simulink model "PVarray_Grid_IncCondReg_det"  (Simulink 8.3)
settings: Solver=FixedStepDiscrete  SolverMode=SingleTasking  StartTime=0.0  StopTime=0.5  RelTol=1e-3
PreLoadFcn:
  | Ts_Power=1e-6
  | Ts_Control=100e-6
undefined symbols (not defined in the file): D1, Delta, DiscIntNeverNeededParam, level, sigbuilder_block
libraries: powerlib x30, powerlib_extras x8, simulink x4
(part 2 of 2)

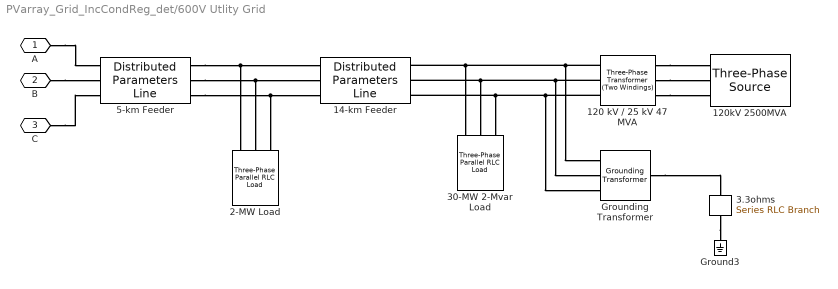
== system PVarray_Grid_IncCondReg_det/600V Utlity Grid ==
  120 kV / 25 kV 47 MVA : powerlib/Elements/Three-Phase Transformer (Two Windings)  Winding1Connection=Yg  UNITS=pu  NominalPower=[47e6 60 ]  Winding1="[ 120e3  0.08/30   0.08 ]"  Winding2Connection=Delta (D1)  Winding2="[ 25e3  0.08/30  0.08]"  SetSaturation=off  Rm=500  Lm=500  Saturation="[ 0,0  ;  0.005,1.2  ;  1.0,1.4 ]"  Hysteresis=off  DataFile='basic_model'  SetInitialFlux=off  InitialFluxes=[ 0.8 , -0.8 , 0.7 ]  Measurements=None  MoreParameters=off  BreakLoop=off  DataType=off  TransfoNumber=0
  120kV 2500MVA : powerlib/Electrical Sources/Three-Phase Source  Voltage=120e3  PhaseAngle=0  Frequency=60  InternalConnection=Yg  SpecifyImpedance=on  Resistance=0.8929  Inductance=16.58e-3  ShortCircuitLevel=2500e6  BaseVoltage=120e3  XRratio=7  BusType=swing  Pref=0  Qref=0  Qmin=-inf  Qmax=inf
  14-km Feeder : powerlib/Elements/Distributed Parameters Line  Phases=3  Frequency=60  Resistance=[0.1153 0.413]  Inductance=[1.05e-3 3.32e-3]  Capacitance=[11.33e-009 5.01e-009]  Length=14  x1=[-5.8e-05 1.17635592444979e-09 0 0;-5.7e-05 1.1770598483649e-09 0 0;-5.6e-05 1.17776360499355e-09 0 0;-5.5e-05 1.17846719423573e-09 0 0;-5.4e-05 1.17917061599144e-09 0 0;-5.3e-05 1.17987387016071e-09 0 0;-5.2e-05 1.18057695664358e-09 0 0;-5.1e-05 1.18127987534014e-09 0 0;-5e-05 1.18198262615049e-09 0 0;-4.9e-05 1.18268520897475e-09 -3790.50088209165 -24060.9143986541;-4.8e-05 1.18338762371306e-09 -3781.42986191954 -24062.3416739909;-4.7e-05 1.1840898702656e-09 -3772.35830432192 -24063.7655295324;-4.6e-05 1.18479194853256e-09 -3763.28621058805 -24065.1859650761;-4.5e-05 1.18549385841416e-09 -3754.21358200728 -24066.6029804202;-4.4e-05 1.18619559981065e-09 -3745.14041986903 -24068.0165753633;-4.3e-05 1.18689717262229e-09 -3736.06672546281 -24069.4267497044;-4.2e-05 1.18759857674937e-09 -3726.99250007819 -24070.8335032433;-4.1e-05 1.1882998120922e-09 -3717.91774500481 -24072.2368357798;-4e-05 1.18900087855114e-09 -3708.84246153241 -24073.6367471147;-3.9e-05 1.18970177602653e-09 -3699.76665095078 -24075.0332370489;-3.8e-05 1.19040250441876e-09 -3690.6903145498 -24076.426305384;-3.7e-05 1.19110306362825e-09 -3681.61345361941 -24077.8159519219;-3.6e-05 1.19180345355544e-09 -3672.53606944965 -24079.2021764653;-3.5e-05 1.19250367410077e-09 -3663.45816333061 -24080.584978817;-3.4e-05 1.19320372516474e-09 -3654.37973655246 -24081.9643587805;-3.3e-05 1.19390360664784e-09 -3645.30079040545 -24083.3403161598;-3.2e-05 1.19460331845062e-09 -3636.22132617991 -24084.7128507594;-3.1e-05 1.19530286047362e-09 -3627.14134516621 -24086.0819623841;-3e-05 1.19600223261744e-09 -3618.06084865485 -24087.4476508394;-2.9e-05 1.19670143478266e-09 -3608.97983793634 -24088.8099159313;-2.8e-05 1.19740046686991e-09 -3599.89831430132 -24090.168757466;-2.7e-05 1.19809932877986e-09 -3590.81627904046 -24091.5241752505;-2.6e-05 1.19879802041318e-09 -3581.73373344453 -24092.8761690921;-2.5e-05 1.19949654167056e-09 -3572.65067880435 -24094.2247387987;-2.4e-05 1.20019489245273e-09 -3563.56711641084 -24095.5698841786;-2.3e-05 1.20089307266044e-09 -3554.48304755497 -24096.9116050407;-2.2e-05 1.20159108219446e-09 -3545.39847352778 -24098.2499011942;-2.1e-05 1.20228892095559e-09 -3536.3133956204 -24099.584772449;-2e-05 1.20298658884465e-09 -3527.22781512403 -24100.9162186153;-1.9e-05 1.20368408576249e-09 -3518.14173332992 -24102.244239504;-1.8e-05 1.20438141160998e-09 -3509.0551515294 -24103.5688349262;-1.7e-05 1.20507856628801e-09 -3499.96807101389 -24104.8900046937;-1.6e-05 1.2057755496975e-09 -3490.88049307487 -24106.2077486188;-1.5e-05 1.20647236173939e-09 -3481.79241900387 -24107.5220665142;-1.4e-05 1.20716900231466e-09 -3472.70385009252 -24108.832958193;-1.3e-05 1.20786547132428e-09 -3463.61478763251 -24110.140423469;-1.2e-05 1.20856176866929e-09 -3454.52523291559 -24111.4444621563;-1.1e-05 1.20925789425071e-09 -3445.43518723359 -24112.7450740697;-1e-05 1.20995384796962e-09 -3436.34465187842 -24114.0422590242;-9e-06 1.21064962972711e-09 -3427.25362814203 -24115.3360168356;-8e-06 1.21134523942428e-09 -3418.16211731647 -24116.6263473199;-7e-06 1.21204067696228e-09 -3409.07012069384 -24117.9132502937;-6e-06 1.21273594224227e-09 -3399.97763956632 -24119.1967255742;-5e-06 1.21343103516543e-09 -3390.88467522615 -24120.476772979;-4e-06 1.21412595563299e-09 -3381.79122896565 -24121.753392326;-3e-06 1.21482070354617e-09 -3372.69730207719 -24123.026583434;-2e-06 1.21551527880623e-09 -3363.60289585323 -24124.2963461219;-1e-06 1.21620968131446e-09 -3354.50801158628 -24125.5626802092]  x2=[-5.8e-05 1.27313609791547e-09 0 0;-5.7e-05 1.27386533401627e-09 0 0;-5.6e-05 1.27459438907241e-09 0 0;-5.5e-05 1.27532326298026e-09 0 0;-5.4e-05 1.27605195563622e-09 0 0;-5.3e-05 1.27678046693675e-09 0 0;-5.2e-05 1.2775087967783e-09 0 0;-5.1e-05 1.27823694505736e-09 0 0;-5e-05 1.27896491167044e-09 0 0;-4.9e-05 1.27969269651409e-09 -3379.3379853252 -24243.9018981791;-4.8e-05 1.28042029948486e-09 -3370.19800971033 -24245.174155756;-4.7e-05 1.28114772047935e-09 -3361.05755511516 -24246.4429675529;-4.6e-05 1.28187495939418e-09 -3351.91662283875 -24247.7083333896;-4.5e-05 1.28260201612599e-09 -3342.77521418024 -24248.9702530861;-4.4e-05 1.28332889057145e-09 -3333.63333043882 -24250.2287264632;-4.3e-05 1.28405558262726e-09 -3324.49097291376 -24251.483753342;-4.2e-05 1.28478209219012e-09 -3315.34814290439 -24252.735333544;-4.1e-05 1.28550841915681e-09 -3306.20484171011 -24253.9834668915;-4e-05 1.28623456342407e-09 -3297.06107063039 -24255.228153207;-3.9e-05 1.28696052488872e-09 -3287.91683096476 -24256.4693923137;-3.8e-05 1.28768630344758e-09 -3278.77212401283 -24257.7071840352;-3.7e-05 1.28841189899749e-09 -3269.62695107425 -24258.9415281954;-3.6e-05 1.28913731143534e-09 -3260.48131344876 -24260.172424619;-3.5e-05 1.28986254065803e-09 -3251.33521243617 -24261.3998731311;-3.4e-05 1.29058758656249e-09 -3242.18864933633 -24262.6238735572;-3.3e-05 1.29131244904567e-09 -3233.04162544918 -24263.8444257234;-3.2e-05 1.29203712800455e-09 -3223.89414207471 -24265.0615294561;-3.1e-05 1.29276162333614e-09 -3214.74620051298 -24266.2751845825;-3e-05 1.29348593493747e-09 -3205.59780206413 -24267.4853909299;-2.9e-05 1.2942100627056e-09 -3196.44894802833 -24268.6921483265;-2.8e-05 1.29493400653762e-09 -3187.29963970586 -24269.8954566007;-2.7e-05 1.29565776633064e-09 -3178.14987839702 -24271.0953155815;-2.6e-05 1.2963813419818e-09 -3168.99966540221 -24272.2917250983;-2.5e-05 1.29710473338825e-09 -3159.84900202187 -24273.4846849812;-2.4e-05 1.2978279404472e-09 -3150.69788955652 -24274.6741950606;-2.3e-05 1.29855096305585e-09 -3141.54632930674 -24275.8602551674;-2.2e-05 1.29927380111145e-09 -3132.39432257315 -24277.042865133;-2.1e-05 1.29999645451126e-09 -3123.24187065648 -24278.2220247895;-2e-05 1.30071892315259e-09 -3114.08897485748 -24279.3977339692;-1.9e-05 1.30144120693275e-09 -3104.93563647699 -24280.5699925049;-1.8e-05 1.30216330574909e-09 -3095.78185681591 -24281.7388002302;-1.7e-05 1.30288521949899e-09 -3086.62763717517 -24282.9041569789;-1.6e-05 1.30360694807983e-09 -3077.47297885582 -24284.0660625853;-1.5e-05 1.30432849138906e-09 -3068.31788315892 -24285.2245168844;-1.4e-05 1.30504984932412e-09 -3059.16235138562 -24286.3795197115;-1.3e-05 1.3057710217825e-09 -3050.00638483713 -24287.5310709024;-1.2e-05 1.30649200866169e-09 -3040.84998481471 -24288.6791702935;-1.1e-05 1.30721280985922e-09 -3031.69315261969 -24289.8238177216;-1e-05 1.30793342527267e-09 -3022.53588955346 -24290.965013024;-9e-06 1.3086538547996e-09 -3013.37819691747 -24292.1027560386;-8e-06 1.30937409833764e-09 -3004.22007601324 -24293.2370466037;-7e-06 1.31009415578442e-09 -2995.06152814233 -24294.3678845579;-6e-06 1.3108140270376e-09 -2985.90255460639 -24295.4952697407;-5e-06 1.31153371199487e-09 -2976.74315670711 -24296.6192019918;-4e-06 1.31225321055396e-09 -2967.58333574623 -24297.7396811514;-3e-06 1.31297252261259e-09 -2958.42309302558 -24298.8567070603;-2e-06 1.31369164806855e-09 -2949.26242984704 -24299.9702795598;-1e-06 1.31441058681963e-09 -2940.10134751252 -24301.0803984916]  x3=[-5.8e-05 -2.75037560687932e-13 0 0;-5.7e-05 -2.71761263610655e-13 0 0;-5.6e-05 -2.68484927910041e-13 0 0;-5.5e-05 -2.65208554051731e-13 0 0;-5.4e-05 -2.61932142501371e-13 0 0;-5.3e-05 -2.58655693724612e-13 0 0;-5.2e-05 -2.55379208187111e-13 0 0;-5.1e-05 -2.52102686354528e-13 0 0;-5e-05 -2.48826128692532e-13 0 0;-4.9e-05 -2.45549535666793e-13 -23.6102100345883 -155.666879550902;-4.8e-05 -2.4227290774299e-13 -23.5515233271852 -155.675769328311;-4.7e-05 -2.38996245386803e-13 -23.4928332725853 -155.684636980721;-4.6e-05 -2.35719549063919e-13 -23.43413987913 -155.693482506872;-4.5e-05 -2.32442819240031e-13 -23.3754431551607 -155.702305905508;-4.4e-05 -2.29166056380834e-13 -23.3167431090196 -155.711107175373;-4.3e-05 -2.2588926095203e-13 -23.2580397490494 -155.719886315217;-4.2e-05 -2.22612433419324e-13 -23.199333083593 -155.728643323792;-4.1e-05 -2.19335574248427e-13 -23.140623120994 -155.737378199855;-4e-05 -2.16058683905053e-13 -23.0819098695963 -155.746090942162;-3.9e-05 -2.12781762854921e-13 -23.0231933377445 -155.754781549477;-3.8e-05 -2.09504811563756e-13 -22.9644735337835 -155.763450020564;-3.7e-05 -2.06227830497284e-13 -22.9057504660586 -155.77209635419;-3.6e-05 -2.02950820121239e-13 -22.8470241429158 -155.780720549128;-3.5e-05 -1.99673780901356e-13 -22.7882945727013 -155.789322604151;-3.4e-05 -1.96396713303376e-13 -22.7295617637619 -155.797902518037;-3.3e-05 -1.93119617793042e-13 -22.6708257244449 -155.806460289567;-3.2e-05 -1.89842494836105e-13 -22.612086463098 -155.814995917523;-3.1e-05 -1.86565344898314e-13 -22.5533439880693 -155.823509400694;-3e-05 -1.83288168445428e-13 -22.4945983077074 -155.832000737869;-2.9e-05 -1.80010965943205e-13 -22.4358494303615 -155.840469927842;-2.8e-05 -1.7673373785741e-13 -22.3770973643809 -155.848916969408;-2.7e-05 -1.73456484653808e-13 -22.3183421181158 -155.857341861368;-2.6e-05 -1.70179206798172e-13 -22.2595836999166 -155.865744602523;-2.5e-05 -1.66901904756276e-13 -22.200822118134 -155.87412519168;-2.4e-05 -1.63624578993896e-13 -22.1420573811196 -155.882483627647;-2.3e-05 -1.60347229976815e-13 -22.083289497225 -155.890819909237;-2.2e-05 -1.57069858170816e-13 -22.0245184748024 -155.899134035265;-2.1e-05 -1.53792464041688e-13 -21.9657443222046 -155.907426004549;-2e-05 -1.5051504805522e-13 -21.9069670477846 -155.915695815911;-1.9e-05 -1.47237610677208e-13 -21.8481866598961 -155.923943468176;-1.8e-05 -1.43960152373447e-13 -21.789403166893 -155.93216896017;-1.7e-05 -1.40682673609739e-13 -21.7306165771297 -155.940372290726;-1.6e-05 -1.37405174851884e-13 -21.6718268989613 -155.948553458677;-1.5e-05 -1.3412765656569e-13 -21.6130341407428 -155.956712462861;-1.4e-05 -1.30850119216965e-13 -21.5542383108303 -155.964849302118;-1.3e-05 -1.2757256327152e-13 -21.4954394175798 -155.972963975292;-1.2e-05 -1.24294989195168e-13 -21.4366374693479 -155.981056481229;-1.1e-05 -1.21017397453727e-13 -21.3778324744918 -155.989126818779;-1e-05 -1.17739788513014e-13 -21.3190244413689 -155.997174986795;-9e-06 -1.14462162838852e-13 -21.2602133783372 -156.005200984134;-8e-06 -1.11184520897063e-13 -21.2013992937551 -156.013204809655;-7e-06 -1.07906863153475e-13 -21.1425821959813 -156.02118646222;-6e-06 -1.04629190073915e-13 -21.083762093375 -156.029145940694;-5e-06 -1.01351502124213e-13 -21.0249389942959 -156.037083243948;-4e-06 -9.80737997702028e-14 -20.9661129071042 -156.044998370852;-3e-06 -9.47960834777184e-14 -20.9072838401601 -156.052891320281;-2e-06 -9.15183537125964e-14 -20.8484518018248 -156.060762091115;-1e-06 -8.82406109406753e-14 -20.7896168004596 -156.068610682234]  x4=[-5.8e-05 3.5411822113335e-12 0 0;-5.7e-05 3.53990398331012e-12 0 0;-5.6e-05 3.53862525218744e-12 0 0;-5.5e-05 3.53734601814719e-12 0 0;-5.4e-05 3.53606628137119e-12 0 0;-5.3e-05 3.53478604204131e-12 0 0;-5.2e-05 3.53350530033949e-12 0 0;-5.1e-05 3.53222405644777e-12 0 0;-5e-05 3.53094231054824e-12 0 0;-4.9e-05 3.52966006282306e-12 -1.28892375629158 -2.1654706090284;-4.8e-05 3.52837731345447e-12 -1.28810730153168 -2.16595636794452;-4.7e-05 3.52709406262477e-12 -1.28729066370301 -2.16644181902993;-4.6e-05 3.52581031051635e-12 -1.28647384292163 -2.16692696221564;-4.5e-05 3.52452605731165e-12 -1.28565683930363 -2.16741179743271;-4.4e-05 3.52324130319319e-12 -1.28483965296511 -2.16789632461222;-4.3e-05 3.52195604834357e-12 -1.28402228402223 -2.16838054368532;-4.2e-05 3.52067029294545e-12 -1.28320473259114 -2.16886445458318;-4.1e-05 3.51938403718157e-12 -1.28238699878805 -2.16934805723704;-4e-05 3.51809728123472e-12 -1.28156908272916 -2.16983135157815;-3.9e-05 3.5168100252878e-12 -1.28075098453072 -2.17031433753784;-3.8e-05 3.51552226952373e-12 -1.27993270430901 -2.17079701504747;-3.7e-05 3.51423401412555e-12 -1.27911424218031 -2.17127938403842;-3.6e-05 3.51294525927635e-12 -1.27829559826096 -2.17176144444215;-3.5e-05 3.51165600515927e-12 -1.27747677266729 -2.17224319619014;-3.4e-05 3.51036625195756e-12 -1.27665776551568 -2.17272463921393;-3.3e-05 3.50907599985453e-12 -1.27583857692254 -2.1732057734451;-3.2e-05 3.50778524903353e-12 -1.27501920700427 -2.17368659881526;-3.1e-05 3.50649399967802e-12 -1.27419965587735 -2.17416711525607;-3e-05 3.50520225197151e-12 -1.27337992365823 -2.17464732269925;-2.9e-05 3.50391000609759e-12 -1.27256001046343 -2.17512722107655;-2.8e-05 3.50261726223992e-12 -1.27173991640947 -2.17560681031976;-2.7e-05 3.50132402058221e-12 -1.27091964161291 -2.17608609036072;-2.6e-05 3.50003028130828e-12 -1.27009918619032 -2.17656506113132;-2.5e-05 3.49873604460199e-12 -1.26927855025831 -2.17704372256348;-2.4e-05 3.49744131064728e-12 -1.26845773393352 -2.17752207458918;-2.3e-05 3.49614607962816e-12 -1.26763673733259 -2.17800011714043;-2.2e-05 3.49485035172872e-12 -1.26681556057221 -2.17847785014929;-2.1e-05 3.49355412713309e-12 -1.26599420376909 -2.17895527354786;-2e-05 3.49225740602552e-12 -1.26517266703995 -2.1794323872683;-1.9e-05 3.49096018859028e-12 -1.26435095050157 -2.17990919124279;-1.8e-05 3.48966247501174e-12 -1.26352905427072 -2.18038568540356;-1.7e-05 3.48836426547434e-12 -1.26270697846421 -2.1808618696829;-1.6e-05 3.48706556016259e-12 -1.26188472319888 -2.18133774401314;-1.5e-05 3.48576635926105e-12 -1.26106228859158 -2.18181330832663;-1.4e-05 3.48446666295437e-12 -1.26023967475922 -2.1822885625558;-1.3e-05 3.48316647142727e-12 -1.25941688181868 -2.18276350663309;-1.2e-05 3.48186578486453e-12 -1.25859390988693 -2.183238140491;-1.1e-05 3.48056460345102e-12 -1.25777075908091 -2.18371246406209;-1e-05 3.47926292737165e-12 -1.25694742951761 -2.18418647727894;-9e-06 3.47796075681142e-12 -1.25612392131405 -2.18466018007417;-8e-06 3.47665809195541e-12 -1.25530023458727 -2.18513357238048;-7e-06 3.47535493298875e-12 -1.25447636945433 -2.18560665413057;-6e-06 3.47405128009665e-12 -1.25365232603233 -2.18607942525721;-5e-06 3.47274713346438e-12 -1.25282810443836 -2.18655188569321;-4e-06 3.47144249327729e-12 -1.25200370478959 -2.18702403537143;-3e-06 3.47013735972081e-12 -1.25117912720316 -2.18749587422476;-2e-06 3.46883173298042e-12 -1.25035437179628 -2.18796740218613;-1e-06 3.46752561324168e-12 -1.24952943868616 -2.18843861918855]  x5=5.70973484498186e-05  V1=ones(3,3)  V2=ones(3,3)  I1=ones(3,3)  I2=ones(3,3)  nHarmo=1  Measurements=None
  2-MW Load : powerlib/Elements/Three-Phase Parallel RLC Load  LConnTagsString=A|B|C  Configuration=Y (grounded)  NominalVoltage=25e3  NominalFrequency=60  ActivePower=2e6  InductivePower=0  CapacitivePower=0  Measurements=None  LoadType=constant Z
  "3.3ohms " : powerlib/Elements/Series RLC Branch  LConnTagsString=__new0  RConnTagsString=__new0  BranchType=R  Resistance=3.3  Inductance=[]  SetiL0=off  InitialCurrent=0  Capacitance=[]  Setx0=off  InitialVoltage=0  Measurements=None
  30-MW 2-Mvar Load : powerlib/Elements/Three-Phase Parallel RLC Load  LConnTagsString=A|B|C  Configuration=Y (grounded)  NominalVoltage=25e3  NominalFrequency=60  ActivePower=30e6  InductivePower=2e6  CapacitivePower=0  Measurements=None  LoadType=constant Z
  5-km Feeder : powerlib/Elements/Distributed Parameters Line  Phases=3  Frequency=60  Resistance=[0.1153 0.413]  Inductance=[1.05e-3 3.32e-3]  Capacitance=[11.33e-009 5.01e-009]  Length=5  x1=[-2.1e-05 1.20806252804395e-09 -3536.88834563418 -24100.7824567799;-2e-05 1.2087451259397e-09 -3527.8023135806 -24102.1141196122;-1.9e-05 1.2094275520458e-09 -3518.71578014764 -24103.4423569965;-1.8e-05 1.21010980626528e-09 -3509.62874662669 -24104.7671687441;-1.7e-05 1.21079188850117e-09 -3500.54121430922 -24106.0885546668;-1.6e-05 1.21147379865653e-09 -3491.45318448679 -24107.4065145766;-1.5e-05 1.21215553663444e-09 -3482.36465845099 -24108.7210482863;-1.4e-05 1.21283710233802e-09 -3473.2756374935 -24110.0321556092;-1.3e-05 1.2135184956704e-09 -3464.18612290609 -24111.3398363587;-1.2e-05 1.21419971653473e-09 -3455.09611598058 -24112.6440903491;-1.1e-05 1.21488076483421e-09 -3446.00561800885 -24113.9449173951;-1e-05 1.21556164047204e-09 -3436.91463028287 -24115.2423173117;-9e-06 1.21624234335145e-09 -3427.82315409468 -24116.5362899146;-8e-06 1.21692287337569e-09 -3418.73119073637 -24117.8268350198;-7e-06 1.21760323044806e-09 -3409.63874150011 -24119.1139524439;-6e-06 1.21828341447186e-09 -3400.54580767814 -24120.3976420041;-5e-06 1.21896342535041e-09 -3391.45239056278 -24121.6779035178;-4e-06 1.21964326298707e-09 -3382.3584914464 -24122.9547368032;-3e-06 1.22032292728523e-09 -3373.26411162145 -24124.2281416787;-2e-06 1.22100241814828e-09 -3364.16925238043 -24125.4981179633;-1e-06 1.22168173547966e-09 -3355.07391501594 -24126.7646654767]  x2=[-2.1e-05 1.20229252106794e-09 -3536.3133956204 -24099.584772449;-2e-05 1.20299001752641e-09 -3527.22781512403 -24100.9162186153;-1.9e-05 1.20368734301318e-09 -3518.14173332992 -24102.244239504;-1.8e-05 1.20438449742912e-09 -3509.0551515294 -24103.5688349262;-1.7e-05 1.20508148067517e-09 -3499.96807101389 -24104.8900046937;-1.6e-05 1.20577829265226e-09 -3490.88049307487 -24106.2077486188;-1.5e-05 1.20647493326137e-09 -3481.79241900387 -24107.5220665142;-1.4e-05 1.20717140240349e-09 -3472.70385009252 -24108.832958193;-1.3e-05 1.20786769997962e-09 -3463.61478763251 -24110.140423469;-1.2e-05 1.20856382589082e-09 -3454.52523291559 -24111.4444621563;-1.1e-05 1.20925978003815e-09 -3445.43518723359 -24112.7450740697;-1e-05 1.20995556232269e-09 -3436.34465187842 -24114.0422590242;-9e-06 1.21065117264556e-09 -3427.25362814203 -24115.3360168356;-8e-06 1.2113466109079e-09 -3418.16211731647 -24116.6263473199;-7e-06 1.21204187701088e-09 -3409.07012069384 -24117.9132502937;-6e-06 1.21273697085567e-09 -3399.97763956632 -24119.1967255742;-5e-06 1.21343189234349e-09 -3390.88467522615 -24120.476772979;-4e-06 1.21412664137558e-09 -3381.79122896565 -24121.753392326;-3e-06 1.21482121785319e-09 -3372.69730207719 -24123.026583434;-2e-06 1.21551562167762e-09 -3363.60289585323 -24124.2963461219;-1e-06 1.21620985275017e-09 -3354.50801158628 -24125.5626802092]  x3=[-2.1e-05 -5.47175931720412e-12 -11.2236902755025 -79.1234381044711;-2e-05 -5.47039543674378e-12 -11.1938606452157 -79.1276637133182;-1.9e-05 -5.46903077881825e-12 -11.1640294240315 -79.1318780763596;-1.8e-05 -5.46766534362147e-12 -11.1341966161899 -79.1360811929963;-1.7e-05 -5.46629913134751e-12 -11.1043622259305 -79.1402730626311;-1.6e-05 -5.46493214219054e-12 -11.0745262574937 -79.1444536846681;-1.5e-05 -5.46356437634483e-12 -11.0446887151197 -79.1486230585131;-1.4e-05 -5.46219583400478e-12 -11.0148496030491 -79.1527811835737;-1.3e-05 -5.46082651536489e-12 -10.9850089255227 -79.1569280592588;-1.2e-05 -5.45945642061976e-12 -10.9551666867816 -79.1610636849791;-1.1e-05 -5.45808554996412e-12 -10.925322891067 -79.1651880601468;-1e-05 -5.45671390359279e-12 -10.8954775426203 -79.1693011841758;-9e-06 -5.45534148170073e-12 -10.8656306456833 -79.1734030564815;-8e-06 -5.45396828448298e-12 -10.8357822044978 -79.1774936764809;-7e-06 -5.4525943121347e-12 -10.8059322233061 -79.1815730435927;-6e-06 -5.45121956485117e-12 -10.7760807063504 -79.1856411572371;-5e-06 -5.44984404282777e-12 -10.7462276578733 -79.1896980168358;-4e-06 -5.44846774625999e-12 -10.7163730821175 -79.1937436218124;-3e-06 -5.44709067534343e-12 -10.6865169833262 -79.1977779715919;-2e-06 -5.44571283027381e-12 -10.6566593657425 -79.2018010656009;-1e-06 -5.44433421124695e-12 -10.6268002336098 -79.2058129032677]  x4=[-2.1e-05 6.27481598923702e-12 -12.4922083172085 -78.9091123636864;-2e-05 6.27542552843402e-12 -12.462459395678 -78.9138162077877;-1.9e-05 6.2760341757531e-12 -12.4327087029542 -78.9185088364758;-1.8e-05 6.27664193110776e-12 -12.4029562432652 -78.9231902490838;-1.7e-05 6.27724879441162e-12 -12.3732020208395 -78.9278604449463;-1.6e-05 6.27785476557843e-12 -12.3434460399059 -78.9325194233996;-1.5e-05 6.27845984452208e-12 -12.3136883046932 -78.9371671837816;-1.4e-05 6.27906403115655e-12 -12.2839288194309 -78.9418037254317;-1.3e-05 6.279667325396e-12 -12.2541675883483 -78.9464290476909;-1.2e-05 6.28026972715467e-12 -12.2244046156753 -78.951043149902;-1.1e-05 6.28087123634696e-12 -12.1946399056417 -78.9556460314091;-1e-05 6.28147185288736e-12 -12.1648734624778 -78.960237691558;-9e-06 6.28207157669053e-12 -12.1351052904141 -78.9648181296962;-8e-06 6.28267040767123e-12 -12.1053353936813 -78.9693873451727;-7e-06 6.28326834574435e-12 -12.0755637765104 -78.9739453373381;-6e-06 6.28386539082491e-12 -12.0457904431325 -78.9784921055446;-5e-06 6.28446154282805e-12 -12.0160153977792 -78.9830276491461;-4e-06 6.28505680166906e-12 -11.9862386446821 -78.9875519674978;-3e-06 6.28565116726333e-12 -11.9564601880732 -78.9920650599569;-2e-06 6.28624463952638e-12 -11.9266800321847 -78.9965669258818;-1e-06 6.28683721837388e-12 -11.8968981812489 -79.0010575646329]  x5=2.03919101606495e-05  V1=ones(3,3)  V2=ones(3,3)  I1=ones(3,3)  I2=ones(3,3)  nHarmo=1  Measurements=None
  Ground3 : powerlib/Elements/Ground  LConnTagsString=a
  "Grounding Transformer " : powerlib/Elements/Grounding Transformer   UNITS=pu  NominalPower="[100e6   60]"  NominalVoltage=25e3  ZeroSequenceImpedance_pu=[0.025 0.75]  MagnetizationBranch_pu=[500 500]  ZeroSequenceImpedance_SI=[0.052083 589.05]  MagnetizationBranch_SI=[1041.7 3.927e+005]  Measurements=None
  A : PMIOPort  Port=1  Side=Left
  B : PMIOPort  Port=2  Side=Left
  C : PMIOPort  Port=3  Side=Left
  connections:
  "3.3ohms "/RConn1 -- Ground3/LConn1
  120 kV / 25 kV 47 MVA/LConn1 -- 120kV 2500MVA/RConn1
  120 kV / 25 kV 47 MVA/LConn2 -- 120kV 2500MVA/RConn2
  120 kV / 25 kV 47 MVA/LConn3 -- 120kV 2500MVA/RConn3
  120 kV / 25 kV 47 MVA/RConn1 -- "Grounding Transformer "/LConn1 -- 14-km Feeder/RConn1 -- 30-MW 2-Mvar Load/LConn1
  120 kV / 25 kV 47 MVA/RConn2 -- "Grounding Transformer "/LConn2 -- 14-km Feeder/RConn2 -- 30-MW 2-Mvar Load/LConn2
  120 kV / 25 kV 47 MVA/RConn3 -- "Grounding Transformer "/LConn3 -- 14-km Feeder/RConn3 -- 30-MW 2-Mvar Load/LConn3
  5-km Feeder/RConn1 -- 14-km Feeder/LConn1 -- 2-MW Load/LConn1
  5-km Feeder/RConn2 -- 14-km Feeder/LConn2 -- 2-MW Load/LConn2
  5-km Feeder/RConn3 -- 14-km Feeder/LConn3 -- 2-MW Load/LConn3
  A/RConn1 -- 5-km Feeder/LConn1
  B/RConn1 -- 5-km Feeder/LConn2
  C/RConn1 -- 5-km Feeder/LConn3
  "Grounding Transformer "/RConn1 -- "3.3ohms "/LConn1

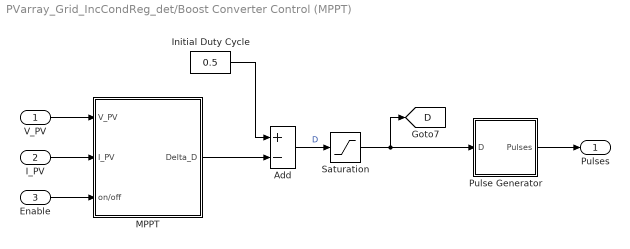
== system PVarray_Grid_IncCondReg_det/Boost Converter Control (MPPT) ==
  V_PV : Inport
  I_PV : Inport  Port=2
  Enable : Inport  Port=3
  Add : Sum  Inputs=+-
  Initial Duty Cycle : Constant  Value=0.5
  MPPT : Subsystem
  Pulse Generator : Subsystem  mask{Freq=5000}
      mask prompts: Freq "Frequency (Hz)"
  Saturation : Saturate  UpperLimit=1  LowerLimit=0
  Pulses : Outport
  tag scope: D=global
  wires:
  Initial Duty Cycle/1 -> Add/1
  MPPT/1(Delta_D) -> Add/2
  Add/1 -> Saturation/1  "D"
  Saturation/1 -> Pulse Generator/1(D), [D]
  Enable/1 -> MPPT/3(on/off)
  Pulse Generator/1(Pulses) -> Pulses/1
  I_PV/1 -> MPPT/2(I_PV)
  V_PV/1 -> MPPT/1(V_PV)

== system PVarray_Grid_IncCondReg_det/Irradiance (W/m2)  ==
  Demux : Demux  Tag=STV Demux  Outputs=1
  FromWs : FromWorkspace  Tag=STV FromWs  VariableName=tuvar  SampleTime=0  SigBuilderData=DataTag0  VnvData=DataTag1
      SigBuilderData=|
      | common.afterFinalStr = 'Extrapolate'
      | common.sampleTime = '0'
      | dataSet(1).timeRange = [0 1]
      | dataSet(1).name = 'Constant Irradiance'
      | dataSet(2).timeRange = [0 1]
      | dataSet(2).name = 'Step Irradiance'
      | dataSet(3).timeRange = [0 3]
      | dataSet(3).name = 'Ramp-up/down Irradiance'
      | sbobj.Groups(1).Name = 'Constant Irradiance'
      | sbobj.Groups(1).Signals.Name = 'Ir'
      | sbobj.Groups(1).Signals.XData = [0 1]
      | sbobj.Groups(1).Signals.YData = [1000 1000]
      | sbobj.Groups(1).TimeRange = [0 1]
      | sbobj.Groups(2).Name = 'Step Irradiance'
      | sbobj.Groups(2).Signals.Name = 'Ir'
      | sbobj.Groups(2).Signals.XData = [0 0.501 0.51 0.69 0.7 1]
      | sbobj.Groups(2).Signals.YData = [1000 1000 250 250 1000 1000]
      | sbobj.Groups(2).TimeRange = [0 1]
      | sbobj.Groups(3).Name = 'Ramp-up/down Irradiance'
      | sbobj.Groups(3).Signals.Name = 'Ir'
      | sbobj.Groups(3).Signals.XData = [0 0.1 0.2 0.3 0.4 0.5 0.6 0.7 0.8 0.9 1 1.1 1.2 1.3 1.4 1.5 1.6 1.7 1.8 1.9 2 2.1 2.2 2.3 2.4 2.5 2.6 2.7 2.8 2.9 3]
      | sbobj.Groups(3).Signals.YData = [1097.75228944 1094.10970969 1097.06246402 1091.52073756 1088.79871699 1125.25999692 1116.55497593 1103.07535159 1087.42881641 1091.34531969 1098.23465886 1107.91416062 1086.67995579 1076.70132844 1085.50902707 1103.33510833 1103.91353604 1104.51679419 1098.69715347 1101.83689096 1095.23846983 1108.62021612 1086.38305529 1104.55029556 1091.5129062 1096.65113061 1105.52783346 1110.39090654 1088.82361317 1112.60658709 1106.60143141]
      | sbobj.Groups(3).TimeRange = [0 3]
  Ir : Outport  Tag=STV Outport
  wires:
  Demux/1 -> Ir/1
  FromWs/1 -> Demux/1

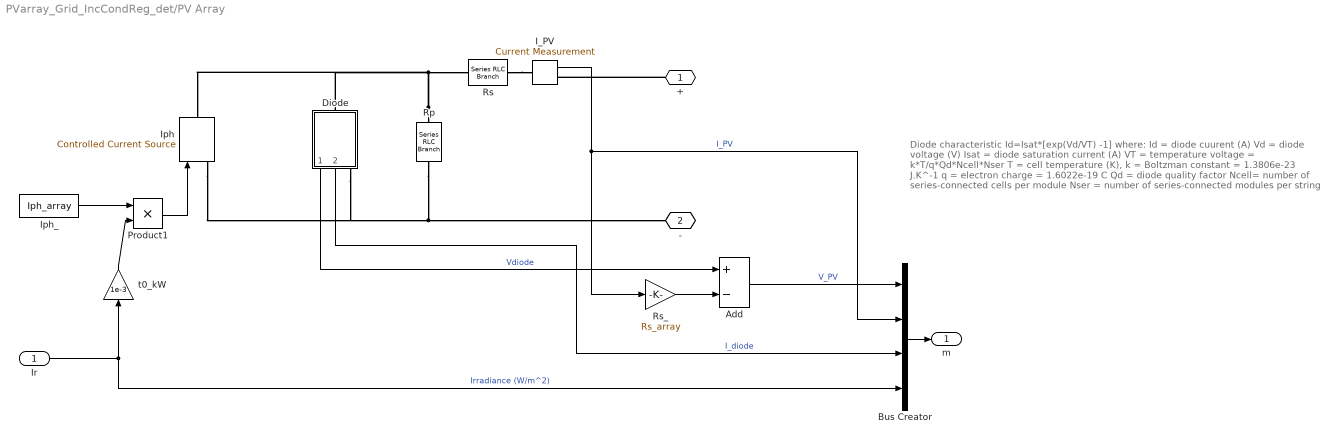
== system PVarray_Grid_IncCondReg_det/PV Array ==
  note: Diode characteristic
      |    Id=Isat*[exp(Vd/VT) -1]
      |
      | where:
      |    Id = diode cuurent (A)
      |    Vd = diode voltage (V)
      |  Isat = diode saturation current (A)
      |    VT = temperature voltage = k*T/q*Qd*Ncell*Nser
      |
      |     T = cell temperature (K),
      |     k = Boltzman constant = 1.3806e-23 J.K^-1
      |     q = electron charge = 1.6022e-19 C
      |    Qd = diode quality factor
      |  Ncell= number of series-connected cells per module
      |  Nser = number of series-connected modules per string
  Ir : Inport
  Add : Sum  Inputs=+-
  Bus Creator : BusCreator
  Diode : Subsystem
      mask Display:
      | plot(-75,-50,100,150, [-15 -15 43 -15 -15 -75],[50 8 50 92 50 50], ...
      |     [43 43],[8 94],[100 43], [50 50])
  I_PV : powerlib/Measurements/Current Measurement  PhasorSimulation=off  OutputType=Complex  PSBequivalent=0
  Iph : powerlib/Electrical Sources/Controlled Current Source  Initialize=on  Source_Type=AC  Amplitude=0  Phase=0  Frequency=0  Measurements=None
  Iph_ : Constant  Value=Iph_array
  Product1 : Product  Inputs=**  RndMeth=Zero
  Rp : powerlib/Elements/Series RLC Branch  LConnTagsString=__new0  RConnTagsString=__new0  BranchType=R  Resistance=Rp_array  Inductance=1e-3  SetiL0=off  InitialCurrent=0  Capacitance=1e-6  Setx0=off  InitialVoltage=0  Measurements=Branch current
  Rs : powerlib/Elements/Series RLC Branch  LConnTagsString=__new0  RConnTagsString=__new0  BranchType=R  Resistance=Rs_array  Inductance=1e-3  SetiL0=off  InitialCurrent=0  Capacitance=1e-6  Setx0=off  InitialVoltage=0  Measurements=None
  Rs_ : Gain  Gain=Rs_array
  t0_kW : Gain  Gain=1e-3
  + : PMIOPort  Port=1  Side=Right
  - : PMIOPort  Port=2  Side=Right
  m : Outport
  wires:
  Bus Creator/1 -> m/1
  Diode/2(Idiode) -> Bus Creator/3  "I_diode"
  Add/1 -> Bus Creator/1  "V_PV"
  t0_kW/1 -> Product1/2
  I_PV/1 -> Bus Creator/2, Rs_/1  "I_PV"
  Rs_/1 -> Add/2
  Diode/1(Vdiode) -> Add/1  "Vdiode"
  Ir/1 -> Bus Creator/4, t0_kW/1  "Irradiance (W/m^2)"
  Iph_/1 -> Product1/1
  Product1/1 -> Iph/1
  connections:
  +/RConn1 -- I_PV/RConn1
  Rs/LConn1 -- I_PV/LConn1
  Rp/LConn1 -- Rs/RConn1 -- Iph/RConn1 -- Diode/LConn1
  Rp/RConn1 -- -/RConn1 -- Diode/RConn1 -- Iph/LConn1

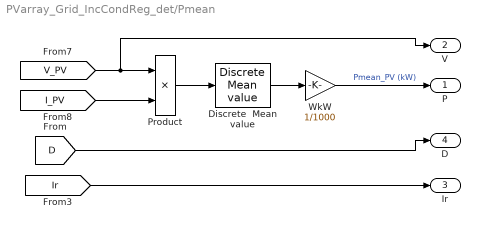
== system PVarray_Grid_IncCondReg_det/Pmean ==
  Discrete  Mean value : powerlib_extras/Discrete Measurements/Discrete  Mean value  Freq=60  Vinit=0  Ts=Ts_Control
  Product : Product  RndMeth=Zero
  WkW : Gain  Gain=1/1000
  P : Outport
  V : Outport  Port=2
  Ir : Outport  Port=3
  D : Outport  Port=4
  wires:
  [V_PV] -> V/1, Product/1
  Product/1 -> Discrete  Mean value/1
  [I_PV] -> Product/2
  WkW/1 -> P/1  "Pmean_PV (kW)"
  Discrete  Mean value/1 -> WkW/1
  [Ir] -> Ir/1
  [D] -> D/1

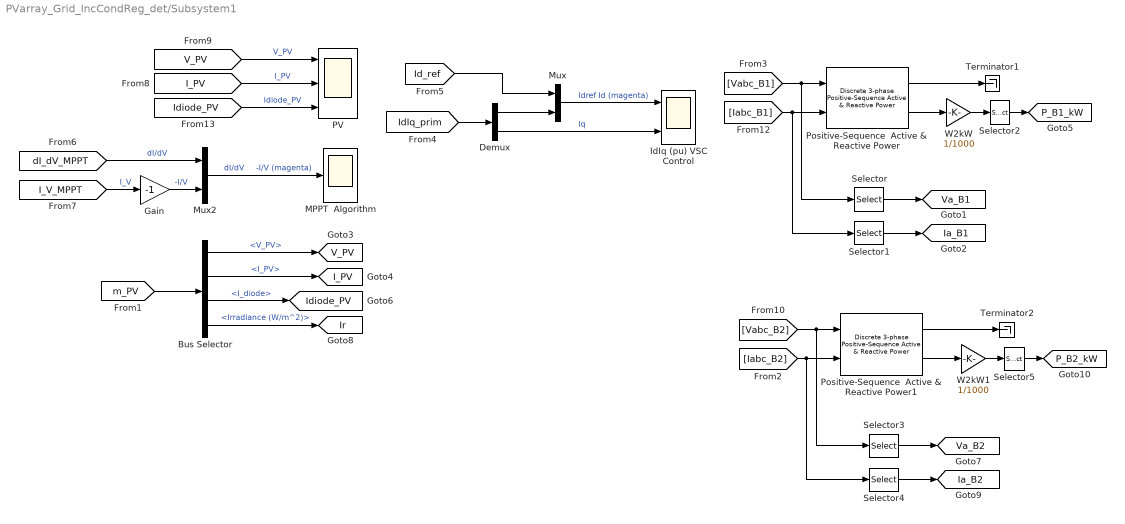
== system PVarray_Grid_IncCondReg_det/Subsystem1 ==
  Bus Selector : BusSelector  OutputSignals=V_PV,I_PV,I_diode,Irradiance (W/m^2)
  Demux : Demux  Outputs=2
  Gain : Gain  Gain=-1
  IdIq (pu) VSC Control : Scope  NumInputPorts=2
      settings: TimeRange=2  YMin=-0.5~-0.5  YMax=1.5~1.5  SaveName=ScopeData8  Decimation=100
  MPPT  Algorithm : Scope
      settings: TimeRange=2  YMin=-2  YMax=0  SaveName=ScopeData6  Decimation=100
  Mux : Mux  Inputs=2
  Mux2 : Mux  Inputs=2
  PV : Scope  NumInputPorts=3
      settings: TimeRange=2  YMin=240~0~0  YMax=280~400~50  SaveName=ScopeData2  Decimation=100
  Positive-Sequence  Active & Reactive Power : powerlib_extras/Discrete Measurements/Discrete 3-phase  Positive-Sequence  Active & Reactive Power  Freq=60  Par_Vinit=[0 0]  Par_Iinit=[0 0]  Ts=Ts_Control
  Positive-Sequence  Active & Reactive Power1 : powerlib_extras/Discrete Measurements/Discrete 3-phase  Positive-Sequence  Active & Reactive Power  Freq=60  Par_Vinit=[0 0]  Par_Iinit=[0 0]  Ts=Ts_Control
  Selector{,1,3..4} (4 alike) : Selector  InputPortWidth=3  Indices=[1]
  Selector2 : Selector  InputPortWidth=2  Indices=[1]
  Selector5 : Selector  InputPortWidth=2  Indices=[1]
  Terminator1 : Terminator
  Terminator2 : Terminator
  W2kW : Gain  Gain=1/1000
  W2kW1 : Gain  Gain=1/1000
  tag scope: I_PV=global, Ia_B1=global, Ia_B2=global, Idiode_PV=global, Ir=global, P_B1_kW=global, P_B2_kW=global, V_PV=global, Va_B1=global, Va_B2=global
  wires:
  [Vabc_B1] -> Positive-Sequence  Active & Reactive Power/1, Selector/1
  [Iabc_B1] -> Positive-Sequence  Active & Reactive Power/2, Selector1/1
  Positive-Sequence  Active & Reactive Power/2 -> W2kW/1
  Positive-Sequence  Active & Reactive Power/1 -> Terminator1/1
  W2kW/1 -> Selector2/1
  [I_V_MPPT] -> Gain/1  "I_V"
  [IdIq_prim] -> Demux/1
  [Id_ref] -> Mux/1
  Demux/1 -> Mux/2
  Mux/1 -> IdIq (pu) VSC Control/1  "Idref Id (magenta)"
  Demux/2 -> IdIq (pu) VSC Control/2  "Iq"
  Selector/1 -> [Va_B1]
  Selector1/1 -> [Ia_B1]
  [V_PV] -> PV/1  "V_PV"
  [I_PV] -> PV/2  "I_PV"
  [Idiode_PV] -> PV/3  "Idiode_PV"
  [dI_dV_MPPT] -> Mux2/1  "dI/dV"
  Gain/1 -> Mux2/2  "-I/V"
  Mux2/1 -> MPPT  Algorithm/1  "dI/dV     -I/V (magenta)"
  Selector2/1 -> [P_B1_kW]
  [m_PV] -> Bus Selector/1
  Bus Selector/1 -> [V_PV]  "<V_PV>"
  Bus Selector/2 -> [I_PV]  "<I_PV>"
  Bus Selector/3 -> [Idiode_PV]  "<I_diode>"
  Bus Selector/4 -> [Ir]  "<Irradiance (W/m^2)>"
  [Vabc_B2] -> Positive-Sequence  Active & Reactive Power1/1, Selector3/1
  [Iabc_B2] -> Positive-Sequence  Active & Reactive Power1/2, Selector4/1
  Positive-Sequence  Active & Reactive Power1/2 -> W2kW1/1
  Positive-Sequence  Active & Reactive Power1/1 -> Terminator2/1
  W2kW1/1 -> Selector5/1
  Selector3/1 -> [Va_B2]
  Selector4/1 -> [Ia_B2]
  Selector5/1 -> [P_B2_kW]

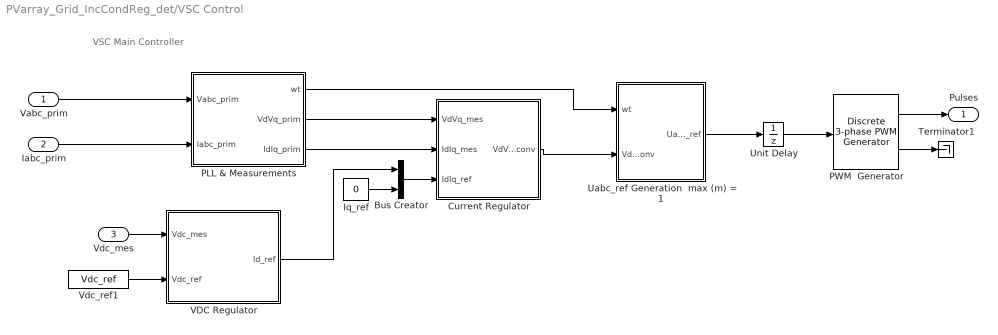
== system PVarray_Grid_IncCondReg_det/VSC Control ==
  note: VSC Main Controller
  Vabc_prim : Inport  PortDimensions=3
  Iabc_prim : Inport  Port=2  PortDimensions=3
  Vdc_mes : Inport  Port=3  PortDimensions=1
  Bus Creator : BusCreator  Inputs=2
  Current Regulator : Subsystem
  Iq_ref : Constant  Value=0
  PLL & Measurements : Subsystem
  PWM  Generator : powerlib_extras/Discrete  Control Blocks/Discrete 3-phase PWM Generator  ModulatorType=3-level  ModulatorMode=Un-synchronized  nF=18  Fc=33*60  ModulatingSignals=off  m=0.2  Freq=60  Phase=0  Ts=Ts_Power
  Terminator1 : Terminator
  Uabc_ref Generation  max (m) = 1 : Subsystem
  Unit Delay : UnitDelay  SampleTime=Ts_Control
  VDC Regulator : Subsystem
  Vdc_ref1 : Constant  Value=Vdc_ref
  Pulses : Outport
  wires:
  VDC Regulator/1(Id_ref) -> Bus Creator/1
  PLL & Measurements/1(wt) -> Uabc_ref Generation  max (m) = 1/1(wt)
  Current Regulator/1(VdVq_conv) -> Uabc_ref Generation  max (m) = 1/2(VdVq_conv)
  Iq_ref/1 -> Bus Creator/2
  Bus Creator/1 -> Current Regulator/3(IdIq_ref)
  PLL & Measurements/3(IdIq_prim) -> Current Regulator/2(IdIq_mes)
  PLL & Measurements/2(VdVq_prim) -> Current Regulator/1(VdVq_mes)
  Vdc_mes/1 -> VDC Regulator/1(Vdc_mes)
  Vabc_prim/1 -> PLL & Measurements/1(Vabc_prim)
  Iabc_prim/1 -> PLL & Measurements/2(Iabc_prim)
  Unit Delay/1 -> PWM  Generator/1
  PWM  Generator/1 -> Pulses/1
  Uabc_ref Generation  max (m) = 1/1(Uabc_ref) -> Unit Delay/1
  PWM  Generator/2 -> Terminator1/1
  Vdc_ref1/1 -> VDC Regulator/2(Vdc_ref)

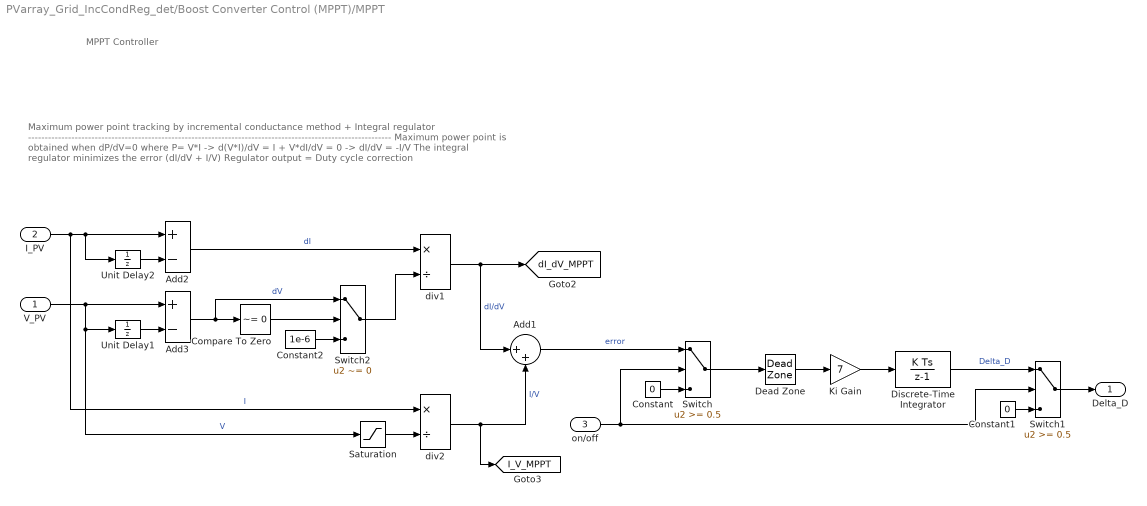
== system PVarray_Grid_IncCondReg_det/Boost Converter Control (MPPT)/MPPT ==
  note: Maximum power point tracking by incremental conductance method + Integral regulator
      | -------------------------------------------------------------------------------------------------------------
      | Maximum power point is obtained when dP/dV=0  where P= V*I
      | -> d(V*I)/dV = I + V*dI/dV = 0
      | -> dI/dV = -I/V
      | The integral regulator minimizes the error (dI/dV + I/V)
      | Regulator output = Duty cycle correction
  note: MPPT Controller
  V_PV : Inport
  I_PV : Inport  Port=2
  on/off : Inport  Port=3
  Add1 : Sum  Inputs=|++
  Add2 : Sum  Inputs=+-
  Add3 : Sum  Inputs=+-
  Compare To Zero : simulink/Logic and Bit Operations/Compare To Zero  relop=~=  OutDataTypeStr=uint8
  Constant : Constant  Value=0
  Constant1 : Constant  Value=0
  Constant2 : Constant  Value=1e-6
  Dead Zone : DeadZone  LowerValue=-0.02  UpperValue=+0.02  SaturateOnIntegerOverflow=on
  Discrete-Time Integrator : DiscreteIntegrator  gainval=1  SampleTime=Ts_Control  LimitOutput=on  UpperSaturationLimit=1  LowerSaturationLimit=-1  ICPrevOutput=DiscIntNeverNeededParam  ICPrevScaledInput=DiscIntNeverNeededParam
  Ki Gain : Gain  Gain=7
  Saturation : Saturate  UpperLimit=inf  LowerLimit=eps
  Switch : Switch  Threshold=0.5
  Switch1 : Switch  Threshold=0.5
  Switch2 : Switch  Criteria=u2 ~= 0
  Unit Delay1 : UnitDelay  SampleTime=Ts_Control
  Unit Delay2 : UnitDelay  SampleTime=Ts_Control
  div1 : Product  Inputs=*/  RndMeth=Zero
  div2 : Product  Inputs=*/  RndMeth=Zero
  Delta_D : Outport
  tag scope: I_V_MPPT=global, dI_dV_MPPT=global
  wires:
  V_PV/1 -> Add3/1, Saturation/1, Unit Delay1/1  "V"
  div1/1 -> [dI_dV_MPPT], Add1/1  "dI/dV"
  Constant/1 -> Switch/3
  Switch/1 -> Dead Zone/1
  Unit Delay1/1 -> Add3/2
  Compare To Zero/1 -> Switch2/2
  Switch2/1 -> div1/2
  Constant2/1 -> Switch2/3
  I_PV/1 -> Unit Delay2/1, Add2/1, div2/1  "I"
  Unit Delay2/1 -> Add2/2
  Add3/1 -> Compare To Zero/1, Switch2/1  "dV"
  Add2/1 -> div1/1  "dI"
  Saturation/1 -> div2/2
  div2/1 -> Add1/2, [I_V_MPPT]  "I/V"
  Add1/1 -> Switch/1  "error"
  Dead Zone/1 -> Ki Gain/1
  Constant1/1 -> Switch1/3
  Discrete-Time Integrator/1 -> Switch1/1  "Delta_D"
  Switch1/1 -> Delta_D/1
  on/off/1 -> Switch/2, Switch1/2
  Ki Gain/1 -> Discrete-Time Integrator/1

== system PVarray_Grid_IncCondReg_det/Boost Converter Control (MPPT)/Pulse Generator ==
  D : Inport
  Relational Operator : RelationalOperator  Operator=<=  OutDataTypeStr=boolean
  Repeating Sequence : simulink/Sources/Repeating Sequence  rep_seq_t="[0  1/Freq]"  rep_seq_y=[0 1]
  Pulses : Outport
  wires:
  D/1 -> Relational Operator/2
  Relational Operator/1 -> Pulses/1
  Repeating Sequence/1 -> Relational Operator/1

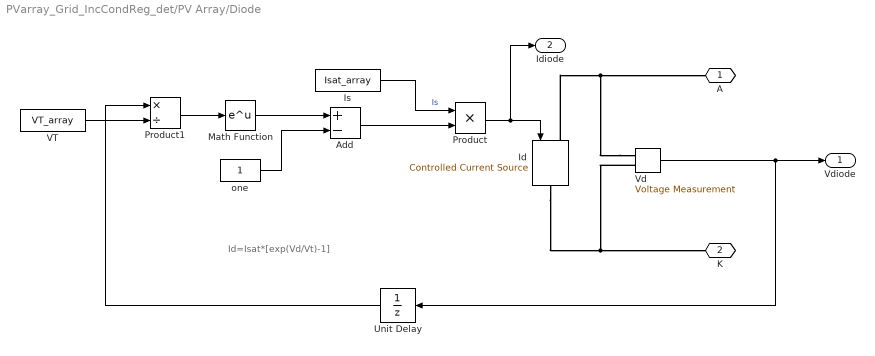
== system PVarray_Grid_IncCondReg_det/PV Array/Diode ==
  note: Id=Isat*[exp(Vd/Vt)-1]
  Add : Sum  Inputs=+-
  Id : powerlib/Electrical Sources/Controlled Current Source  Initialize=on  Source_Type=AC  Amplitude=0  Phase=0  Frequency=0  Measurements=None
  Is : Constant  Value=Isat_array
  Math Function : Math  SaturateOnIntegerOverflow=on
  Product : Product  RndMeth=Zero
  Product1 : Product  Inputs=*/  RndMeth=Zero
  Unit Delay : UnitDelay  SampleTime=Ts
  VT : Constant  Value=VT_array
  Vd : powerlib/Measurements/Voltage Measurement  PhasorSimulation=off  OutputType=Complex  PSBequivalent=0
  one : Constant
  A : PMIOPort  Port=1  Side=Left
  K : PMIOPort  Port=2  Side=Right
  Vdiode : Outport
  Idiode : Outport  Port=2
  wires:
  Product/1 -> Idiode/1, Id/1
  Vd/1 -> Vdiode/1, Unit Delay/1
  Is/1 -> Product/1  "Is"
  Product1/1 -> Math Function/1
  one/1 -> Add/2
  Add/1 -> Product/2
  VT/1 -> Product1/2
  Unit Delay/1 -> Product1/1
  Math Function/1 -> Add/1
  connections:
  Id/RConn1 -- K/RConn1 -- Vd/LConn2
  Vd/LConn1 -- A/RConn1 -- Id/LConn1

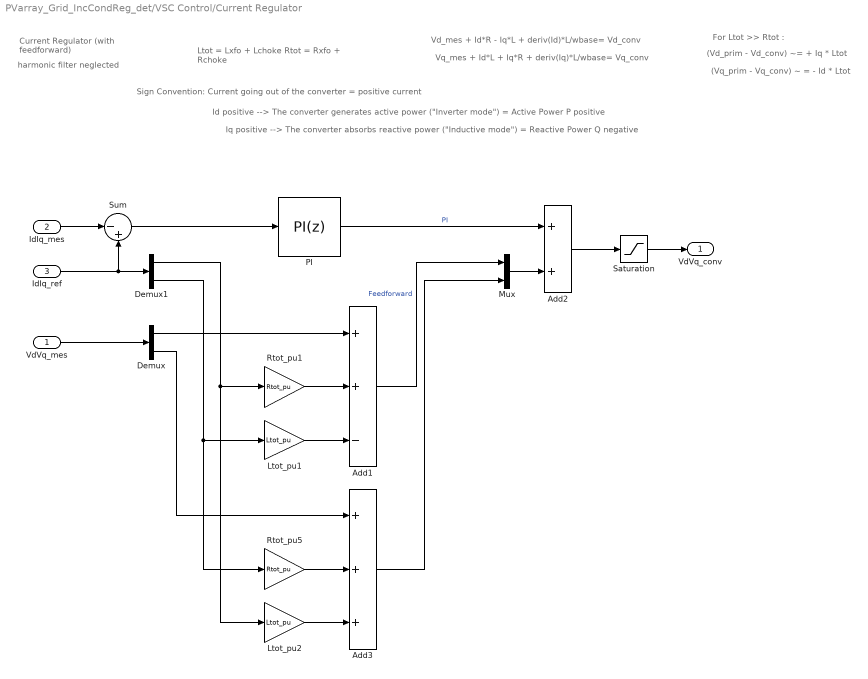
== system PVarray_Grid_IncCondReg_det/VSC Control/Current Regulator ==
  note: harmonic filter neglected
  note: Vd_mes + Id*R - Iq*L + deriv(Id)*L/wbase= Vd_conv
  note: Vq_mes + Id*L + Iq*R + deriv(Iq)*L/wbase= Vq_conv
  note: Current Regulator
      | (with feedforward)
  note: Sign Convention: Current going out of the converter = positive current
  note: Iq positive --> The converter absorbs reactive power ("Inductive mode") = Reactive Power Q negative
  note: Id positive --> The converter generates active power ("Inverter mode") = Active Power P positive
  note: Ltot = Lxfo + Lchoke
      | Rtot = Rxfo + Rchoke
  note: (Vd_prim - Vd_conv) ~= + Iq * Ltot
  note: (Vq_prim - Vq_conv) ~ = - Id * Ltot
  note: For Ltot >> Rtot :
  VdVq_mes : Inport  PortDimensions=2
  IdIq_mes : Inport  Port=2  PortDimensions=2
  IdIq_ref : Inport  Port=3  PortDimensions=2
  Add1 : Sum  Inputs=++-
  Add2 : Sum
  Add3 : Sum  Inputs=+++
  Demux : Demux  Outputs=2
  Demux1 : Demux  Outputs=2
  Ltot_pu1 : Gain  Gain=Ltot_pu  SaturateOnIntegerOverflow=on  OutDataTypeStr=Inherit: Same as input  ParamDataTypeStr=Inherit: Same as input
  Ltot_pu2 : Gain  Gain=Ltot_pu  SaturateOnIntegerOverflow=on  OutDataTypeStr=Inherit: Same as input  ParamDataTypeStr=Inherit: Same as input
  Mux : Mux  Inputs=2
  PI : simulink/Continuous/PID Controller  Controller=PI  TimeDomain=Discrete-time  SampleTime=Ts  IntegratorMethod=Forward Euler  FilterMethod=Forward Euler  Form=Parallel  P=Kp_Ireg  I=Ki_Ireg  D=0  N=100  InitialConditionSource=internal  InitialConditionForIntegrator=0  InitialConditionForFilter=0  ExternalReset=none  LimitOutput=on  UpperSaturationLimit=2  LowerSaturationLimit=-2  LinearizeAsGain=off  AntiWindupMode=none  Kb=1  TrackingMode=off  Kt=1  PParamMin=[]  PParamMax=[]  IParamMin=[]  IParamMax=[]  DParamMin=[]  DParamMax=[]  NParamMin=[]  NParamMax=[]  KbParamMin=[]  KbParamMax=[]  KtParamMin=[]  KtParamMax=[]  POutMin=[]  POutMax=[]  IOutMin=[]  IOutMax=[]  DOutMin=[]  DOutMax=[]  NOutMin=[]  NOutMax=[]  KbOutMin=[]  KbOutMax=[]  KtOutMin=[]  KtOutMax=[]  IntegratorOutMin=[]  IntegratorOutMax=[]  FilterOutMin=[]  FilterOutMax=[]  SumOutMin=[]  SumOutMax=[]  SumI1OutMin=[]  SumI1OutMax=[]  SumI2OutMin=[]  SumI2OutMax=[]  SumI3OutMin=[]  SumI3OutMax=[]  SumDOutMin=[]  SumDOutMax=[]  SaturationOutMin=[]  SaturationOutMax=[]  IntegratorContinuousStateAttributes=''  IntegratorStateMustResolveToSignalObject=off  IntegratorRTWStateStorageClass=Auto  FilterContinuousStateAttributes=''  FilterStateMustResolveToSignalObject=off  FilterRTWStateStorageClass=Auto
  Rtot_pu1 : Gain  Gain=Rtot_pu  SaturateOnIntegerOverflow=on  OutDataTypeStr=Inherit: Same as input  ParamDataTypeStr=Inherit: Same as input
  Rtot_pu5 : Gain  Gain=Rtot_pu  SaturateOnIntegerOverflow=on  OutDataTypeStr=Inherit: Same as input  ParamDataTypeStr=Inherit: Same as input
  Saturation : Saturate  UpperLimit=2  LowerLimit=-2
  Sum : Sum  Inputs=|-+
  VdVq_conv : Outport
  wires:
  Mux/1 -> Add2/2
  PI/1 -> Add2/1  "PI"
  Sum/1 -> PI/1
  IdIq_ref/1 -> Sum/2, Demux1/1
  IdIq_mes/1 -> Sum/1
  Add2/1 -> Saturation/1
  Saturation/1 -> VdVq_conv/1
  VdVq_mes/1 -> Demux/1
  Demux/1 -> Add1/1
  Rtot_pu1/1 -> Add1/2
  Demux1/1 -> Rtot_pu1/1, Ltot_pu2/1
  Ltot_pu1/1 -> Add1/3
  Demux1/2 -> Ltot_pu1/1, Rtot_pu5/1
  Rtot_pu5/1 -> Add3/2
  Ltot_pu2/1 -> Add3/3
  Add1/1 -> Mux/1  "Feedforward"
  Demux/2 -> Add3/1
  Add3/1 -> Mux/2

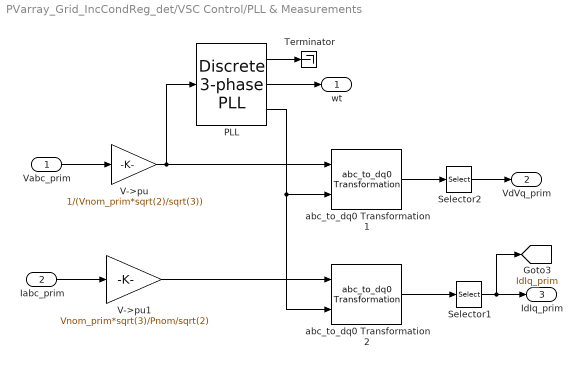
== system PVarray_Grid_IncCondReg_det/VSC Control/PLL & Measurements ==
  Vabc_prim : Inport
  Iabc_prim : Inport  Port=2
  PLL : powerlib_extras/Discrete  Control Blocks/Discrete 3-phase PLL  Fmin=45  Par_Init="[-0.57  Fnom]"  ParK=[60 1400]  Ts=Ts  AGC=off
  Selector1 : Selector  InputPortWidth=3  Indices=[1 2]
  Selector2 : Selector  InputPortWidth=3  Indices=[1 2]
  Terminator : Terminator
  V->pu : Gain  Gain=1/(Vnom_prim*sqrt(2)/sqrt(3))  SaturateOnIntegerOverflow=on  OutDataTypeStr=Inherit: Same as input  ParamDataTypeStr=Inherit: Same as input
  V->pu1 : Gain  Gain=Vnom_prim*sqrt(3)/Pnom/sqrt(2)  SaturateOnIntegerOverflow=on  OutDataTypeStr=Inherit: Same as input  ParamDataTypeStr=Inherit: Same as input
  abc_to_dq0 Transformation1 : powerlib_extras/Measurements/abc_to_dq0 Transformation
  abc_to_dq0 Transformation2 : powerlib_extras/Measurements/abc_to_dq0 Transformation
  wt : Outport
  VdVq_prim : Outport  Port=2
  IdIq_prim : Outport  Port=3
  tag scope: IdIq_prim=global
  wires:
  V->pu1/1 -> abc_to_dq0 Transformation2/1
  V->pu/1 -> abc_to_dq0 Transformation1/1, PLL/1
  abc_to_dq0 Transformation2/1 -> Selector1/1
  PLL/2 -> wt/1
  Vabc_prim/1 -> V->pu/1
  Iabc_prim/1 -> V->pu1/1
  abc_to_dq0 Transformation1/1 -> Selector2/1
  Selector2/1 -> VdVq_prim/1
  Selector1/1 -> [IdIq_prim], IdIq_prim/1
  PLL/3 -> abc_to_dq0 Transformation2/2, abc_to_dq0 Transformation1/2
  PLL/1 -> Terminator/1

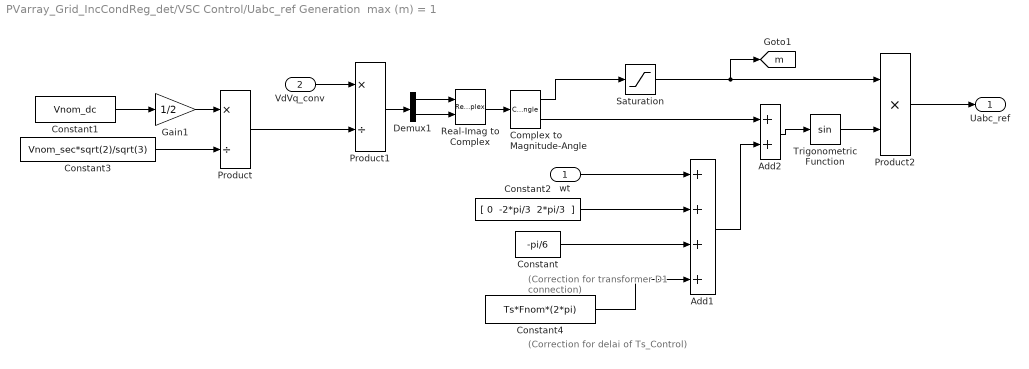
== system PVarray_Grid_IncCondReg_det/VSC Control/Uabc_ref Generation  max (m) = 1 ==
  note: (Correction for transformer
      |  D1 connection)
  note: (Correction for delai of Ts_Control)
  wt : Inport
  VdVq_conv : Inport  Port=2
  Add1 : Sum  Inputs=++++
  Add2 : Sum
  Complex to Magnitude-Angle : ComplexToMagnitudeAngle
  Constant : Constant  Value=-pi/6
  Constant1 : Constant  Value=Vnom_dc
  Constant2 : Constant  Value="[ 0  -2*pi/3  2*pi/3  ]"
  Constant3 : Constant  Value=Vnom_sec*sqrt(2)/sqrt(3)
  Constant4 : Constant  Value=Ts*Fnom*(2*pi)
  Demux1 : Demux  Outputs=2
  Gain1 : Gain  Gain=1/2
  Product : Product  Inputs=*/  RndMeth=Zero
  Product1 : Product  Inputs=*/  RndMeth=Zero
  Product2 : Product  Inputs=**  RndMeth=Zero
  Real-Imag to Complex : RealImagToComplex
  Saturation : Saturate  UpperLimit=1  LowerLimit=0
  Trigonometric Function : Trigonometry
  Uabc_ref : Outport
  tag scope: m=global
  wires:
  Complex to Magnitude-Angle/1 -> Saturation/1
  Constant1/1 -> Gain1/1
  VdVq_conv/1 -> Product1/1
  Product1/1 -> Demux1/1
  Gain1/1 -> Product/1
  Real-Imag to Complex/1 -> Complex to Magnitude-Angle/1
  Demux1/1 -> Real-Imag to Complex/1
  Demux1/2 -> Real-Imag to Complex/2
  Constant2/1 -> Add1/2
  Constant/1 -> Add1/3
  Constant3/1 -> Product/2
  Product/1 -> Product1/2
  Complex to Magnitude-Angle/2 -> Add2/1
  Add1/1 -> Add2/2
  Add2/1 -> Trigonometric Function/1
  Saturation/1 -> [m], Product2/1
  Trigonometric Function/1 -> Product2/2
  Product2/1 -> Uabc_ref/1
  wt/1 -> Add1/1
  Constant4/1 -> Add1/4

== system PVarray_Grid_IncCondReg_det/VSC Control/VDC Regulator ==
  Vdc_mes : Inport  PortDimensions=1
  Vdc_ref : Inport  Port=2  PortDimensions=1
  PI : simulink/Continuous/PID Controller  Controller=PI  TimeDomain=Discrete-time  SampleTime=Ts  IntegratorMethod=Trapezoidal  FilterMethod=Forward Euler  Form=Parallel  P=Kp_VDCreg  I=Ki_VDCreg  D=0  N=100  InitialConditionSource=internal  InitialConditionForIntegrator=0  InitialConditionForFilter=0  ExternalReset=none  LimitOutput=on  UpperSaturationLimit=1.5  LowerSaturationLimit=-1.5  LinearizeAsGain=off  AntiWindupMode=none  Kb=1  TrackingMode=off  Kt=1  PParamMin=[]  PParamMax=[]  IParamMin=[]  IParamMax=[]  DParamMin=[]  DParamMax=[]  NParamMin=[]  NParamMax=[]  KbParamMin=[]  KbParamMax=[]  KtParamMin=[]  KtParamMax=[]  POutMin=[]  POutMax=[]  IOutMin=[]  IOutMax=[]  DOutMin=[]  DOutMax=[]  NOutMin=[]  NOutMax=[]  KbOutMin=[]  KbOutMax=[]  KtOutMin=[]  KtOutMax=[]  IntegratorOutMin=[]  IntegratorOutMax=[]  FilterOutMin=[]  FilterOutMax=[]  SumOutMin=[]  SumOutMax=[]  SumI1OutMin=[]  SumI1OutMax=[]  SumI2OutMin=[]  SumI2OutMax=[]  SumI3OutMin=[]  SumI3OutMax=[]  SumDOutMin=[]  SumDOutMax=[]  SaturationOutMin=[]  SaturationOutMax=[]  IntegratorContinuousStateAttributes=''  IntegratorStateMustResolveToSignalObject=off  IntegratorRTWStateStorageClass=Auto  FilterContinuousStateAttributes=''  FilterStateMustResolveToSignalObject=off  FilterRTWStateStorageClass=Auto
  Rtot_pu3 : Gain  Gain=1/Vnom_dc  SaturateOnIntegerOverflow=on  OutDataTypeStr=Inherit: Same as input  ParamDataTypeStr=Inherit: Same as input
  Sum : Sum  Inputs=|+-
  Id_ref : Outport  SampleTime=Ts  InitialOutput=0
  tag scope: Id_ref=global, Vdc_ref=global
  wires:
  Sum/1 -> Rtot_pu3/1
  Vdc_mes/1 -> Sum/1
  Vdc_ref/1 -> Sum/2, [Vdc_ref]
  Rtot_pu3/1 -> PI/1
  PI/1 -> [Id_ref], Id_ref/1
